simulink model "DemonstratorSimscape"  (R2020b)
settings: Solver=ode113  StartTime=0.0  StopTime=t_stop*0+20  FixedStep=1e-4
values from neighbouring files (symbols this model uses):
  brkD = 0    [main.m]
  brkI = 1e4    (= 10000)    [main.m]
  brkP = 1e5    (= 100000)    [main.m]
  d_drm = 0.5*d_drum    [main.m]
  d_shm = 0.4*d_sheave    [main.m]
  DeltaCable0 = 0    [main.m]
  Droop_scaling = 0    [main.m]
  eta_sh = 0.015    [main.m]
  filt_NUM = ones(1,200)*0.005    [main.m]
  g = 9.80665    [main.m]
  Iw = 0.5*(W.i + M.in*GB.r^2)    [main.m]
  Kp_mul = 0.3    [main.m]
  Lc0 = abs((T.ph-L.height-P.d-L.z0)*0.001)    [main.m]
  Ls1 = ((T.ph-0.5*W.pd)/1000)    [main.m]
  Ls2 = ((0.5*(T.s2+P.d)-2*P.d)/1000)    [main.m]
  M = 50e3    (= 50000)    [calcGrav.m]
  phi0_drm = -90    [main.m]
  phi0_shm = -90    [main.m]
  r_sheave = P.d*0.5    [main.m]
  s = tf('s')    [calcGrav.m]
  tau_brk = 0.001    [main.m]
  tau_em = 60e-3    (= 0.06)    [calcGrav.m]    (also in main.m)
  tau_m = tau_w/GB.r    [main.m]
  Tmax = 400e3    (= 400000)    [main.m]
  Tn_mul = 10    [main.m]
  x_drm = 0.7*r_drum    [main.m]
  x_shm = 0.7*r_sheave    [main.m]
  z0 = 0    [calcGrav.m]    (also in main.m = L.z0-P.d*0.5-P.d-P.d-L.height-T.h1-T.h2-32)
undefined symbols (not defined in the file or in its folder): C, CA, Controller_sampleTime, DiscIntNeverNeededParam, GB, L, P, Part, T, VFD_acceleration_model_factor, VFD_Adapt_factor_lower_p1458, VFD_Adapt_factor_upper_p1459, VFD_Curr_limit_var_p0641, VFD_Current_limit_p0640, VFD_Id_setp_total_r1624, VFD_Iq, VFD_Kp_n_basic_p1460, VFD_M, VFD_M_accel_T_smooth_p1517, VFD_M_lim_var_fixS_src_p1551, VFD_M_max_lower_p1521, VFD_M_max_lower_scal_p1525, VFD_M_max_up_mot_scal_p1524, VFD_M_max_upper_p1520, VFD_n_act_T_smooth_p1442, VFD_n_ctr_Kp_n_up_scal_p1461, VFD_n_ctr_Tn_n_up_sca_p1463, VFD_n_ctrl_adapt_Kp_lower_p1456, VFD_n_ctrl_adapt_Kp_upper_p1457, VFD_n_ctrl_Adpt_sig_Kp_p1455, VFD_n_ctrl_Kp_scal_p1466, VFD_n_ctrl_n_lower_p1464, VFD_n_ctrl_n_upper_p1465, VFD_n_ctrl_Tn_n_lower_p1462, VFD_n_limit_neg_p1086, VFD_n_limit_pos_p1083, VFD_n_limit_setp_p1063, VFD_n_max_p1082, VFD_n_set_filt_1_T_p1416, VFD_P_max_gen_p1531, VFD_P_max_mot_p1530, VFD_PU_I_outp_max_r0289, VFD_RFG_ramp_down_time_p1121, VFD_RFG_ramp_up_time_p1120, VFD_RFG_t_RD_scal_p1139, VFD_RFG_t_RU_scal_p1138, VSD, W, X, Y, Z
libraries: sm_lib x248, nesl_utility x128, simulink x49, pid_lib x4, cstblocks x2, simulink_extras x2
(part 1 of 10)
settings Model: Creator=pawel  LastModifiedBy=Pawel
settings SolverCC: ZeroCrossAlgorithm=Adaptive
settings DataIOCC: ReturnWorkspaceOutputs=off
settings DebuggingCC: IgnoredZcDiagnostic=none  ArithmeticOperatorsInVariantConditions=warning
settings SFSimCC: CustomCodeUndefinedFunction=UseInterfaceOnly
settings ExplorerConfigSet: InternalSimMechanicsExplorerSettings="<ExplorerConfiguration><canonicalview>planar_xy</canonicalview><AnimationSetting><BasePlaybackSpeed>1.0</BasePlaybackSpeed><PlaybackSpeedFactor>1.0</PlaybackSpeedFactor></AnimationSetting><TilePanel><TileInfo><Tiles Columns=\"1\" Count=\"1\" Rows=\"1\"><Column Weight=\"1\"/><Row Weight=\"1\"/><Tile Height=\"1\" Width=\"1\" X=\"0\" Y=\"0\"/></Tiles></TileInfo><SceneInfo><SceneViewer><BGColor><R>0.60000002384185791</R><G>0.60000002384185791</G><B>0.60000002384185791</B></BGColor><Camera><DoPerspective>off</DoPerspective><Position><X>-3.24512344704319666e-08</X><Y>5.10100123372752456</Y><Z>8.85394363287113606</Z></Position><Center><X>-3.24512344704319666e-08</X><Y>5.10100123372752456</Y><Z>2.95815624440365355e-06</Z></Center><Up><X>0</X><Y>1</Y><Z>0</Z></Up><ViewLimDist>1</ViewLimDist><YLim>5.30553002357482928</YLim><XLim>4.55308148188114892</XLim></Camera></SceneViewer></SceneInfo></TilePanel><MechEditorPanel><Cameras/><GfxPanelCameraMap/><VideoCreator><PlaybackSpeedRatio>1.0</PlaybackSpeedRatio><FrameRate>30</FrameRate><VideoFormat>Motion JPEG AVI</VideoFormat><FrameSize>auto</FrameSize></VideoCreator></MechEditorPanel></ExplorerConfiguration>"

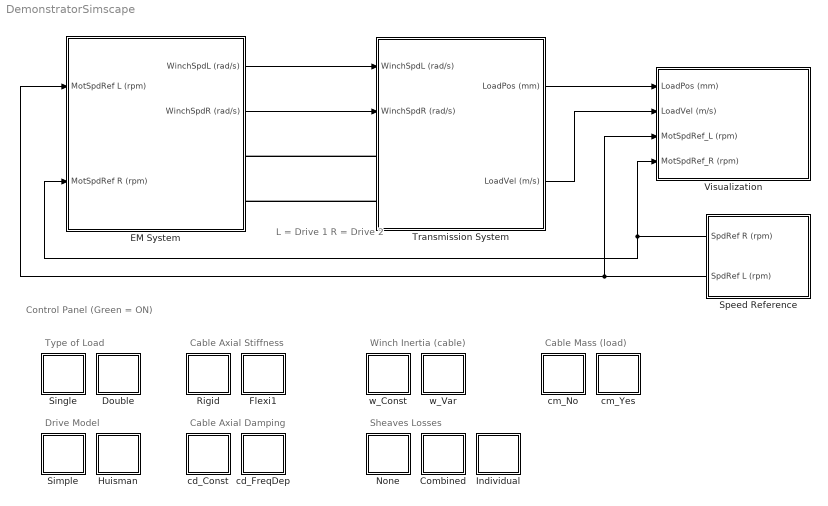
== system DemonstratorSimscape ==
  note: L = Drive 1
      | R = Drive 2
  note: Type of Load
  note: Control Panel (Green = ON)
  note: Cable Axial Stiffness
  note: Sheaves Losses
  note: Cable Mass (load)
  note: Winch Inertia (cable)
  note: Cable Axial Damping
  note: Drive Model
  Combined : Subsystem  Tag=btn_cablelosses
      settings: OpenFcn=cb_switch(gcb)
      mask Display: disp('C')
  Double : Subsystem  Tag=btn_load
      settings: OpenFcn=cb_switch(gcb)
      mask Display: disp('D')
  EM System : Subsystem
  Flexi1 : Subsystem  Tag=btn_cableflex
      settings: OpenFcn=cb_switch(gcb)
      mask Display: disp('F1')
  Huisman : Subsystem  Tag=btn_drive
      settings: OpenFcn=cb_switch(gcb)
      mask Display: disp('H')
  Individual : Subsystem  Tag=btn_cablelosses
      settings: OpenFcn=cb_switch(gcb)
      mask Display: disp('I')
  None : Subsystem  Tag=btn_cablelosses
      settings: OpenFcn=cb_switch(gcb)
      mask Display: disp('N')
  Rigid : Subsystem  Tag=btn_cableflex
      settings: OpenFcn=cb_switch(gcb)
      mask Display: disp('R')
  Simple : Subsystem  Tag=btn_drive
      settings: OpenFcn=cb_switch(gcb)
      mask Display: disp('S')
  Single : Subsystem  Tag=btn_load
      settings: OpenFcn=cb_switch(gcb)
      mask Display: disp('S')
  Speed Reference : Subsystem
  Transmission System : Subsystem
  Visualization : Subsystem
  cd_Const : Subsystem  Tag=btn_cabledamping
      settings: OpenFcn=cb_switch(gcb)
      mask Display: disp('C')
  cd_FreqDep : Subsystem  Tag=btn_cabledamping
      settings: OpenFcn=cb_switch(gcb)
      mask Display: disp('FD')
  cm_No : Subsystem  Tag=btn_cablemass
      settings: OpenFcn=cb_switch(gcb)
      mask Display: disp('NO')
  cm_Yes : Subsystem  Tag=btn_cablemass
      settings: OpenFcn=cb_switch(gcb)
      mask Display: disp('YES')
  w_Const : Subsystem  Tag=btn_winch
      settings: OpenFcn=cb_switch(gcb)
      mask Display: disp('C')
  w_Var : Subsystem  Tag=btn_winch
      settings: OpenFcn=cb_switch(gcb)
      mask Display: disp('V')
  wires:
  EM System/1(WinchSpdL (rad/s)) -> Transmission System/1(WinchSpdL (rad/s))
  EM System/2(WinchSpdR (rad/s)) -> Transmission System/2(WinchSpdR (rad/s))
  Transmission System/1(LoadPos (mm)) -> Visualization/1(LoadPos (mm))
  Transmission System/2(LoadVel (m/s)) -> Visualization/2(LoadVel (m/s))
  Speed Reference/2(SpdRef L (rpm)) -> EM System/1(MotSpdRef L (rpm)), Visualization/3(MotSpdRef_L (rpm))
  Speed Reference/1(SpdRef R (rpm)) -> EM System/2(MotSpdRef R (rpm)), Visualization/4(MotSpdRef_R (rpm))
  connections:
  Transmission System/LConn1 -- EM System/RConn1
  Transmission System/LConn2 -- EM System/RConn2

== system DemonstratorSimscape/Combined ==

== system DemonstratorSimscape/Double ==

== system DemonstratorSimscape/EM System ==
  MotSpdRef L (rpm) : Inport  SampleTime=C.ts
  MotSpdRef R (rpm) : Inport  Port=2  SampleTime=C.ts
  Belt-Cable Spool1 : sm_lib/Belts and Cables/Belt-Cable Spool  PitchRadius=W.d*0.5  PitchRadiusUnits=mm  SenseSpoolAngleA=off  SenseFleetAngleA=off
      settings: SourceProductBaseCode=MS
  Belt-Cable Spool2 : sm_lib/Belts and Cables/Belt-Cable Spool  PitchRadius=W.d*0.5  PitchRadiusUnits=mm  SenseSpoolAngleA=off  SenseFleetAngleA=off
      settings: SourceProductBaseCode=MS
  BrakeL_OFF : FromWorkspace  VariableName=BrakeOffL_inp  Interpolate=off  OutputAfterFinalValue=Holding final value
  BrakeR_OFF : FromWorkspace  VariableName=BrakeOffR_inp  Interpolate=off  OutputAfterFinalValue=Holding final value
  Constant : Constant
  Drives : Subsystem
  Motor Winch Left : Subsystem
  Motor Winch Right : Subsystem
  Product : Product
  Product1 : Product
  Winch Left (yellow) : Subsystem
      mask Display: image('sm_cable_drive_right_angle_winch_IMAGE.png');
  Winch Right (blue) : Subsystem
      mask Display: image('sm_cable_drive_right_angle_winch_IMAGE.png');
  swBrake : ManualSwitch  CurrentSetting=0
  swBrake1 : ManualSwitch
  RWinch : PMIOPort  Side=Right
  LWinch : PMIOPort  Port=2  Side=Right
  WinchSpdL (rad/s) : Outport  VectorParamsAs1DForOutWhenUnconnected=off
  WinchSpdR (rad/s) : Outport  Port=2  VectorParamsAs1DForOutWhenUnconnected=off
  tag scope: BrakeL_OFF=global, BrakeR_OFF=global, MotSpd_L_rpm=global, MotSpd_R_rpm=global, MotTrqRef_L_Nm=global, MotTrqRef_R_Nm=global, MotTrq_L_Nm=global, MotTrq_R_Nm=global
  wires:
  Motor Winch Left/2(theta [deg]) -> Winch Left (yellow)/1(theta winch (deg))
  Winch Right (blue)/1(r_winch (mm)) -> Motor Winch Right/2(winch radius)
  Motor Winch Right/2(theta [deg]) -> Winch Right (blue)/1(theta winch (deg))
  Motor Winch Left/3(WinchSpd (rad/s)) -> WinchSpdL (rad/s)/1
  Motor Winch Right/3(WinchSpd (rad/s)) -> WinchSpdR (rad/s)/1
  Drives/1(TrqRefL (Nm)) -> Motor Winch Left/1(MotTrqRef (Nm)), Product/2
  Motor Winch Right/1(MotSpd (rpm)) -> Drives/4(SpdR (rpm)), [MotSpd_R_rpm]
  Motor Winch Left/1(MotSpd (rpm)) -> Drives/1(SpdL (rpm)), [MotSpd_L_rpm]
  Drives/2(TrqRefR (Nm)) -> Product1/2, Motor Winch Right/1(MotTrqRef (Nm))
  Motor Winch Left/4(MotTrq (Nm)) -> [MotTrq_L_Nm]
  Motor Winch Right/4(MotTrq) -> [MotTrq_R_Nm]
  Winch Left (yellow)/1(r_winch (mm)) -> Motor Winch Left/2(winch radius)
  MotSpdRef L (rpm)/1 -> Drives/2(SpdRefL (rpm))
  MotSpdRef R (rpm)/1 -> Drives/3(SpdRefR (rpm))
  Product/1 -> [MotTrqRef_L_Nm]
  Product1/1 -> [MotTrqRef_R_Nm]
  swBrake/1 -> Motor Winch Left/3(Brake), Product/1, [BrakeL_OFF]
  BrakeL_OFF/1 -> swBrake/1
  Constant/1 -> swBrake1/1, swBrake/2
  BrakeR_OFF/1 -> swBrake1/2
  swBrake1/1 -> [BrakeR_OFF], Motor Winch Right/3(Brake), Product1/1
  connections:
  Belt-Cable Spool1/LConn1 -- Winch Right (blue)/LConn1
  RWinch/RConn1 -- Belt-Cable Spool1/RConn1
  Winch Right (blue)/RConn1 -- Motor Winch Right/RConn1
  Belt-Cable Spool2/LConn1 -- Winch Left (yellow)/LConn1
  Winch Left (yellow)/RConn1 -- Motor Winch Left/RConn1
  LWinch/RConn1 -- Belt-Cable Spool2/RConn1

== system DemonstratorSimscape/Flexi1 ==

== system DemonstratorSimscape/Huisman ==

== system DemonstratorSimscape/Individual ==

== system DemonstratorSimscape/None ==

== system DemonstratorSimscape/Rigid ==

== system DemonstratorSimscape/Simple ==

== system DemonstratorSimscape/Single ==

== system DemonstratorSimscape/Speed Reference ==
  Add : Sum
  Gain : Gain
  Gain1 : Gain
  Manual Switch : ManualSwitch
  Manual Switch1 : ManualSwitch
  SpdRef_L_rpm : FromWorkspace  VariableName=SpdRefL_inp  OutputAfterFinalValue=Holding final value
  SpdRef_R_rpm : FromWorkspace  VariableName=SpdRefR_inp  OutputAfterFinalValue=Holding final value
  Step : Step  After=1000  SampleTime=0
  Step1 : Step  Time=10  After=-1000  SampleTime=0
  SpdRef R (rpm) : Outport  VectorParamsAs1DForOutWhenUnconnected=off
  SpdRef L (rpm) : Outport  Port=2  VectorParamsAs1DForOutWhenUnconnected=off
  wires:
  SpdRef_L_rpm/1 -> Gain/1
  SpdRef_R_rpm/1 -> Gain1/1
  Step1/1 -> Add/2
  Step/1 -> Add/1
  Add/1 -> Manual Switch1/1, Manual Switch/1
  Gain/1 -> Manual Switch/2
  Gain1/1 -> Manual Switch1/2
  Manual Switch1/1 -> SpdRef R (rpm)/1
  Manual Switch/1 -> SpdRef L (rpm)/1

== system DemonstratorSimscape/Transmission System ==
  WinchSpdL (rad/s) : Inport
  WinchSpdR (rad/s) : Inport  Port=2
  Anchor and Load : Subsystem
  Mechanism Configuration1 : sm_lib/Utilities/Mechanism Configuration  UniformGravity=Constant  GravityVector=[0 -g 0]  GravityVectorUnits=m/s^2  GravityUnits=m/s^2  LinearizationDelta=0.001  JointModeTransitionNonlinearIterations=2
  Roof Pulley Set : Subsystem
  Solver Configuration : nesl_utility/Solver Configuration  PhysicalDomain=network_engine_domain  SubClassName=solver  LeftPortType=input  RightPortType=generic  Tones=[]  Harmonics=[]  SimulateNoise=off  Profile=off  UseLocalSampling=off  EnableSwitchedLinearOptims=on  FrequencyDomain=off  UseCCode=off  RelTol=0.001  AbsTol=1e-06  MinStep=1e-09  ToWorkspace=off  RevertToSquareIcSolve=off  NumHomotopyIterations=100  PhasorMode=off  PhasorModeNumHarmonics=1  DoDC=off  ResidualTolerance=1e-09  UseLocalSolver=off  LocalSolverChoice=NE_PARTITIONING_ADVANCER  LocalSolverSampleTime=0.001  DoFixedCost=off  MaxNonlinIter=30  MaxModeIter=2  ComputeImpulses=off  ImpulseIterations=2  LinearAlgebra=auto  EquationFormulation=NE_TIME_EF  DelaysMemoryBudget=10240  AutomaticFiltering=on  FilteringTimeConstant=0.001  PartitionStorageMethod=AS_NEEDED  PartitionMemoryBudget=1024  PartitionMethod=FAST
  Tower structure : Subsystem
  World Frame : sm_lib/Frames and Transforms/World Frame
  RWinch : PMIOPort  Side=Left
  LWinch : PMIOPort  Port=2  Side=Left
  LoadPos (mm) : Outport
  LoadVel (m/s) : Outport  Port=2
  wires:
  Roof Pulley Set/1(w7) -> Anchor and Load/1(w7)
  Roof Pulley Set/2(w6) -> Anchor and Load/2(w6)
  Roof Pulley Set/3(w4) -> Anchor and Load/3(w4)
  Roof Pulley Set/5(w1) -> Anchor and Load/5(w1)
  Anchor and Load/1(LoadPos (mm)) -> LoadPos (mm)/1
  Roof Pulley Set/4(w2) -> Anchor and Load/4(w2)
  Anchor and Load/2(LoadVel (m/s)) -> LoadVel (m/s)/1
  WinchSpdL (rad/s)/1 -> Anchor and Load/6(wL)
  WinchSpdR (rad/s)/1 -> Anchor and Load/7(wR)
  connections:
  Solver Configuration/RConn1 -- Tower structure/LConn1 -- Mechanism Configuration1/RConn1 -- Roof Pulley Set/LConn1 -- World Frame/RConn1
  Roof Pulley Set/RConn2 -- Anchor and Load/LConn3
  Anchor and Load/LConn1 -- Roof Pulley Set/RConn1
  Roof Pulley Set/RConn3 -- Anchor and Load/LConn4
  Roof Pulley Set/RConn5 -- Anchor and Load/LConn5
  Anchor and Load/LConn2 -- Roof Pulley Set/RConn4
  Roof Pulley Set/LConn2 -- RWinch/RConn1
  Roof Pulley Set/LConn3 -- LWinch/RConn1

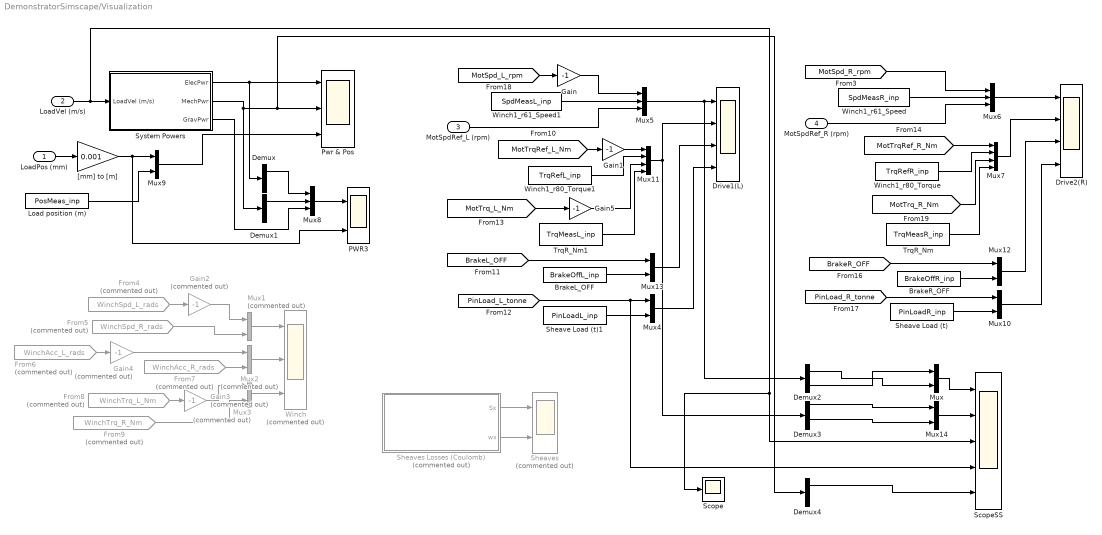
== system DemonstratorSimscape/Visualization ==
  LoadPos (mm) : Inport
  LoadVel (m/s) : Inport  Port=2
  MotSpdRef_L (rpm) : Inport  Port=3
  MotSpdRef_R (rpm) : Inport  Port=4
  BrakeL_OFF : FromWorkspace  VariableName=BrakeOffL_inp  Interpolate=off  OutputAfterFinalValue=Holding final value
  BrakeR_OFF : FromWorkspace  VariableName=BrakeOffR_inp  Interpolate=off  OutputAfterFinalValue=Holding final value
  Demux : Demux  Outputs=2
  Demux1 : Demux  Outputs=2
  Demux2 : Demux  Outputs=3
  Demux3 : Demux
  Demux4 : Demux  Outputs=2
  Drive1(L) : Scope  NumInputPorts=4
  Drive2(R) : Scope  NumInputPorts=4
  From4 : From  Commented=on  GotoTag=WinchSpd_L_rads  TagVisibility=global
  From5 : From  Commented=on  GotoTag=WinchSpd_R_rads  TagVisibility=global
  From6 : From  Commented=on  GotoTag=WinchAcc_L_rads  TagVisibility=global
  From7 : From  Commented=on  GotoTag=WinchAcc_R_rads  TagVisibility=global
  From8 : From  Commented=on  GotoTag=WinchTrq_L_Nm  TagVisibility=global
  From9 : From  Commented=on  GotoTag=WinchTrq_R_Nm  TagVisibility=global
  Gain : Gain  Gain=-1
  Gain1 : Gain  Gain=-1
  Gain2 : Gain  Commented=on  Gain=-1
  Gain3 : Gain  Commented=on  Gain=-1
  Gain4 : Gain  Commented=on  Gain=-1
  Gain5 : Gain  Gain=-1
  Load position (m) : FromWorkspace  VariableName=PosMeas_inp  Interpolate=off  OutputAfterFinalValue=Holding final value
  Mux{,4,9..10,12..14} (7 alike) : Mux  Inputs=2
  Mux1 : Mux  Commented=on  Inputs=2
  Mux11 : Mux
  Mux2 : Mux  Commented=on  Inputs=2
  Mux3 : Mux  Commented=on  Inputs=2
  Mux5 : Mux  Inputs=3
  Mux6 : Mux  Inputs=3
  Mux7 : Mux
  Mux8 : Mux  Inputs=3
  PWR3 : Scope  NumInputPorts=2
  Pwr & Pos : Scope  NumInputPorts=3
  Scope : Scope
  ScopeSS : Scope  NumInputPorts=5
  Sheave Load (t) : FromWorkspace  VariableName=PinLoadR_inp  Interpolate=off  OutputAfterFinalValue=Holding final value
  Sheave Load (t)1 : FromWorkspace  VariableName=PinLoadL_inp  Interpolate=off  OutputAfterFinalValue=Holding final value
  Sheaves : Scope  Commented=on  NumInputPorts=2
  Sheaves Losses (Coulomb) : Subsystem  Commented=on
  System Powers : Subsystem
  TrqR_Nm : FromWorkspace  VariableName=TrqMeasR_inp  OutputAfterFinalValue=Holding final value
  TrqR_Nm1 : FromWorkspace  VariableName=TrqMeasL_inp  OutputAfterFinalValue=Holding final value
  Winch : Scope  Commented=on  NumInputPorts=3
  Winch1_r61_Speed : FromWorkspace  VariableName=SpdMeasR_inp  Interpolate=off  OutputAfterFinalValue=Holding final value
  Winch1_r61_Speed1 : FromWorkspace  VariableName=SpdMeasL_inp  Interpolate=off  OutputAfterFinalValue=Holding final value
  Winch1_r80_Torque : FromWorkspace  VariableName=TrqRefR_inp  Interpolate=off  OutputAfterFinalValue=Holding final value
  Winch1_r80_Torque1 : FromWorkspace  VariableName=TrqRefL_inp  Interpolate=off  OutputAfterFinalValue=Holding final value
  "[mm] to [m]" : Gain  Gain=0.001
  wires:
  Mux1/1 -> Winch/1
  Mux2/1 -> Winch/2
  Mux3/1 -> Winch/3
  From4/1 -> Gain2/1
  From5/1 -> Mux1/2
  From6/1 -> Gain4/1
  From7/1 -> Mux2/2
  From8/1 -> Gain3/1
  From9/1 -> Mux3/2
  Gain2/1 -> Mux1/1
  Gain3/1 -> Mux3/1
  Gain4/1 -> Mux2/1
  "[mm] to [m]"/1 -> PWR3/2, Mux9/1
  MotSpdRef_R (rpm)/1 -> Mux6/3
  [MotTrqRef_R_Nm] -> Mux7/1
  Winch1_r61_Speed/1 -> Mux6/2
  Winch1_r80_Torque/1 -> Mux7/2
  [MotSpd_R_rpm] -> Mux6/1
  Load position (m)/1 -> Mux9/2
  Sheave Load (t)/1 -> Mux10/2
  [PinLoad_R_tonne] -> Mux10/1
  [MotTrq_R_Nm] -> Mux7/3
  TrqR_Nm/1 -> Mux7/4
  Mux6/1 -> Drive2(R)/1
  Mux7/1 -> Drive2(R)/2
  Mux10/1 -> Drive2(R)/4
  Mux4/1 -> Drive1(L)/4
  Mux11/1 -> Demux3/1, Drive1(L)/2
  Mux5/1 -> Demux2/1, Drive1(L)/1
  TrqR_Nm1/1 -> Mux11/4
  [MotTrq_L_Nm] -> Gain5/1
  [PinLoad_L_tonne] -> ScopeSS/4, Mux4/1
  Sheave Load (t)1/1 -> Mux4/2
  [MotSpd_L_rpm] -> Gain/1
  Winch1_r80_Torque1/1 -> Mux11/2
  Winch1_r61_Speed1/1 -> Mux5/2
  [MotTrqRef_L_Nm] -> Gain1/1
  MotSpdRef_L (rpm)/1 -> Mux5/3
  Mux12/1 -> Drive2(R)/3
  Mux13/1 -> Drive1(L)/3
  [BrakeL_OFF] -> Mux13/1
  BrakeL_OFF/1 -> Mux13/2
  [BrakeR_OFF] -> Mux12/1
  BrakeR_OFF/1 -> Mux12/2
  Gain/1 -> Mux5/1
  Gain1/1 -> Mux11/1
  Gain5/1 -> Mux11/3
  LoadPos (mm)/1 -> "[mm] to [m]"/1
  Mux9/1 -> Pwr & Pos/3
  System Powers/1(ElecPwr) -> Demux/1, Pwr & Pos/1
  System Powers/2(MechPwr) -> Demux1/1, Demux4/1, Pwr & Pos/2
  LoadVel (m/s)/1 -> Scope/1, ScopeSS/3, System Powers/1(LoadVel (m/s))
  Mux8/1 -> PWR3/1
  Demux/1 -> Mux8/1
  Demux1/1 -> Mux8/2
  System Powers/3(GravPwr) -> Mux8/3
  Sheaves Losses (Coulomb)/1(Sx) -> Sheaves/1
  Sheaves Losses (Coulomb)/2(wx) -> Sheaves/2
  Mux/1 -> ScopeSS/1
  Mux14/1 -> ScopeSS/2
  Demux4/1 -> ScopeSS/5
  Demux2/3 -> Mux/1
  Demux2/1 -> Mux/2
  Demux3/1 -> Mux14/1
  Demux3/3 -> Mux14/2

== system DemonstratorSimscape/cd_Const ==

== system DemonstratorSimscape/cd_FreqDep ==

== system DemonstratorSimscape/cm_No ==

== system DemonstratorSimscape/cm_Yes ==

== system DemonstratorSimscape/w_Const ==

== system DemonstratorSimscape/w_Var ==

== system DemonstratorSimscape/EM System/Drives ==
  SpdL (rpm) : Inport
  SpdRefL (rpm) : Inport  Port=2
  SpdRefR (rpm) : Inport  Port=3
  SpdR (rpm) : Inport  Port=4
  Add : Sum
  Bus Selector : BusSelector  Commented=on  OutputSignals=signal1.[r1468] Speed Controller P-gain effective,signal1.[r1469] Speed Controller integral time effective,signal1.[r1480] Speed Controller PI torque Output,signal1.[r1481] Speed Controller P torque Output,signal1.[r1482] Speed Controller I torque Output,signal1.[r1508] Torque setpoint before supplementary torque,signal1.[r1516] Supplementary torque and acceleration torque
  Bus Selector1 : BusSelector  Commented=on  OutputSignals=signal1.[r1468] Speed Controller P-gain effective,signal1.[r1469] Speed Controller integral time effective,signal1.[r1480] Speed Controller PI torque Output,signal1.[r1481] Speed Controller P torque Output,signal1.[r1482] Speed Controller I torque Output,signal1.[r1508] Torque setpoint before supplementary torque,signal1.[r1516] Supplementary torque and acceleration torque
  Constant : Constant
  Constant1 : Constant
  DIAG1 : Scope  Commented=on  NumInputPorts=7
  DIAG2 : Scope  Commented=on  NumInputPorts=7
  Gain1 : Gain  Gain=-1
  Gain2 : Gain  Gain=-1
  Gain5 : Gain  Gain=-1
  PLC and Drive Logic Rev3 : Subsystem  AncestorBlock=Control_Library_Rev3/PLC and Drive Logic
  SWTL : ManualSwitch  CurrentSetting=0
  SWTR : ManualSwitch  CurrentSetting=0
  Simple Drive Model : Subsystem  Commented=on
  Simple Drive Model1 : Subsystem  Commented=on
  Step : Step  Time=5  Before=tau_m  After=1.5*tau_m  SampleTime=0
  Step2 : Step  Time=5.2  After=-0.5*tau_m  SampleTime=0
  Winch1_r80_Torque : FromWorkspace  VariableName=TrqRefR_inp  OutputAfterFinalValue=Holding final value
  Winch1_r80_Torque1 : FromWorkspace  VariableName=TrqRefL_inp  OutputAfterFinalValue=Holding final value
  swTrqRefL : ManualSwitch
  swTrqRefR : ManualSwitch
  TrqRefL (Nm) : Outport
  TrqRefR (Nm) : Outport  Port=2
  wires:
  Constant/1 -> PLC and Drive Logic Rev3/3(HMI Motor 1 Start Test [0...1]), PLC and Drive Logic Rev3/5(HMI Motor 2 Start Test [0...1])
  Constant1/1 -> PLC and Drive Logic Rev3/7(WAB Mode)
  SWTL/1 -> swTrqRefL/1
  swTrqRefL/1 -> TrqRefL (Nm)/1
  SWTR/1 -> swTrqRefR/1
  swTrqRefR/1 -> TrqRefR (Nm)/1
  PLC and Drive Logic Rev3/4(M2 [r0079] M_set total (Torque setpoint [Nm])) -> SWTR/2
  Winch1_r80_Torque1/1 -> Gain2/1
  PLC and Drive Logic Rev3/1(M1 [r0079] M_set total (Torque setpoint [Nm])) -> SWTL/2
  Gain5/1 -> PLC and Drive Logic Rev3/8(WAB Motor 1 Speed_Controller Setpoint (r1438))
  SpdL (rpm)/1 -> PLC and Drive Logic Rev3/2(Motor 1 Actual Speed (rpm)), Simple Drive Model/1(Spd_L)
  SpdRefL (rpm)/1 -> Gain5/1, Simple Drive Model/2(SpdRef_L)
  SpdR (rpm)/1 -> PLC and Drive Logic Rev3/6(Motor 2 Actual Speed (rpm)), Simple Drive Model/3(Spd_R)
  SpdRefR (rpm)/1 -> PLC and Drive Logic Rev3/9(WAB Motor 2 Speed_Controller Setpoint (r1438)), Simple Drive Model/4(SpdRef_R)
  Bus Selector/1 -> DIAG1/1  "<[r1468] Speed Controller P-gain effective>"
  Bus Selector/2 -> DIAG1/2  "<[r1469] Speed Controller integral time effective>"
  Bus Selector/3 -> DIAG1/3  "<[r1480] Speed Controller PI torque Output>"
  Bus Selector/4 -> DIAG1/4  "<[r1481] Speed Controller P torque Output>"
  Bus Selector/5 -> DIAG1/5  "<[r1482] Speed Controller I torque Output>"
  Bus Selector/6 -> DIAG1/6  "<[r1508] Torque setpoint before supplementary torque>"
  Bus Selector/7 -> DIAG1/7  "<[r1516] Supplementary torque and acceleration torque>"
  Bus Selector1/1 -> DIAG2/1  "<[r1468] Speed Controller P-gain effective>"
  Bus Selector1/2 -> DIAG2/2  "<[r1469] Speed Controller integral time effective>"
  Bus Selector1/3 -> DIAG2/3  "<[r1480] Speed Controller PI torque Output>"
  Bus Selector1/4 -> DIAG2/4  "<[r1481] Speed Controller P torque Output>"
  Bus Selector1/5 -> DIAG2/5  "<[r1482] Speed Controller I torque Output>"
  Bus Selector1/6 -> DIAG2/6  "<[r1508] Torque setpoint before supplementary torque>"
  Bus Selector1/7 -> DIAG2/7  "<[r1516] Supplementary torque and acceleration torque>"
  PLC and Drive Logic Rev3/3(Motor 1 Diagnostics Bus) -> Bus Selector/1
  PLC and Drive Logic Rev3/5(Motor 2 Diagnostics Bus) -> Bus Selector1/1
  Simple Drive Model/2(TrqSat_R) -> SWTR/1
  Step/1 -> Add/1
  Step2/1 -> Add/2
  Add/1 -> swTrqRefR/2, Gain1/1
  Gain1/1 -> swTrqRefL/2
  Simple Drive Model/1(TrqSat_L) -> SWTL/1

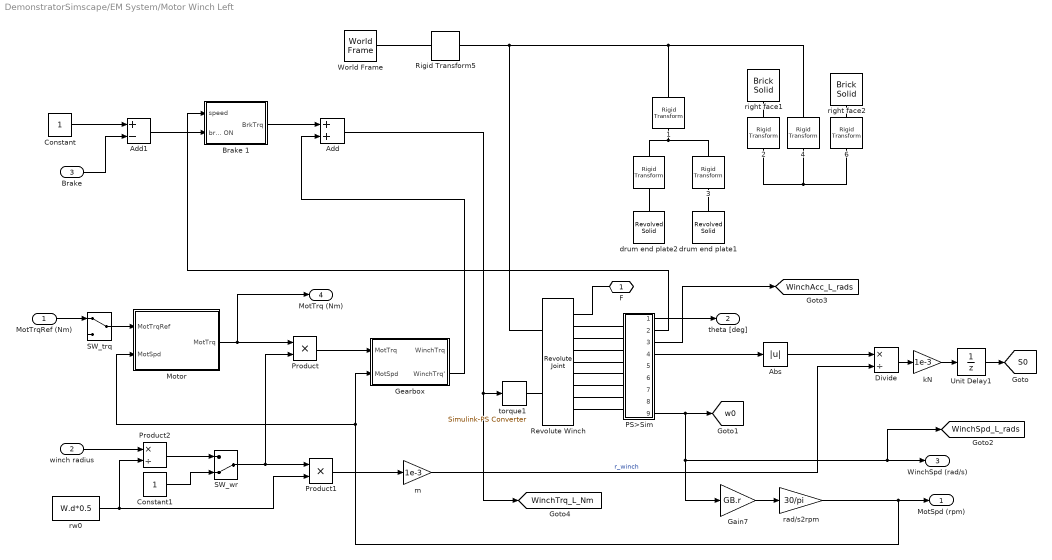
== system DemonstratorSimscape/EM System/Motor Winch Left ==
  MotTrqRef (Nm) : Inport
  winch radius : Inport  Port=2
  Brake : Inport  Port=3
  " " : sm_lib/Frames and Transforms/Rigid Transform  TranslationMethod=Cartesian  TranslationStandardOffset=0  TranslationLengthUnit=mm  TranslationStandardAxis=+Z  TranslationCartesianOffset=[0 0 -W.pds*.5]  TranslationROffset=0  TranslationROffsetUnits=m  TranslationZOffset=0  TranslationZOffsetUnits=m  TranslationThetaOffset=0  TranslationThetaOffsetUnits=deg  RotationMethod=StandardAxis  RotationAngleUnits=deg  RotationStandardAxis=-X  RotationAngle=90  RotationArbitraryAxis=[1 0 0]  FollAlignAxisA=+X  BaseAlignAxisA=+Y  FollAlignAxisB=+Y  BaseAlignAxisB=+Z  RotationSequenceAxes=FollowerAxes  RotationSequence=XYX  RotationSequenceAngles=[0 0 0]  RotationSequenceAnglesUnits=deg  RotationMatrix=[1 0 0; 0 1 0; 0 0 1]
  " 1" : sm_lib/Frames and Transforms/Rigid Transform  TranslationMethod=Cartesian  TranslationStandardOffset=0  TranslationLengthUnit=mm  TranslationStandardAxis=+Z  TranslationCartesianOffset=[0 0 W.w*0.5+W.pds*0.5]  TranslationROffset=0  TranslationROffsetUnits=m  TranslationZOffset=0  TranslationZOffsetUnits=m  TranslationThetaOffset=0  TranslationThetaOffsetUnits=deg  RotationMethod=StandardAxis  RotationAngleUnits=deg  RotationStandardAxis=+X  RotationAngle=90  RotationArbitraryAxis=[1 0 0]  FollAlignAxisA=+X  BaseAlignAxisA=+Y  FollAlignAxisB=+Y  BaseAlignAxisB=+Z  RotationSequenceAxes=FollowerAxes  RotationSequence=XYX  RotationSequenceAngles=[0 0 0]  RotationSequenceAnglesUnits=deg  RotationMatrix=[1 0 0; 0 1 0; 0 0 1]
  " 2" : sm_lib/Frames and Transforms/Rigid Transform  TranslationMethod=Cartesian  TranslationStandardOffset=0  TranslationLengthUnit=mm  TranslationStandardAxis=+Z  TranslationCartesianOffset=[0 -W.pd*.25 -W.pds]  TranslationROffset=0  TranslationROffsetUnits=m  TranslationZOffset=0  TranslationZOffsetUnits=m  TranslationThetaOffset=0  TranslationThetaOffsetUnits=deg  RotationMethod=ArbitraryAxis  RotationAngleUnits=deg  RotationStandardAxis=+X  RotationAngle=90  RotationArbitraryAxis=[1 0 0]  FollAlignAxisA=+X  BaseAlignAxisA=+Y  FollAlignAxisB=+Y  BaseAlignAxisB=+Z  RotationSequenceAxes=FollowerAxes  RotationSequence=XYX  RotationSequenceAngles=[0 0 0]  RotationSequenceAnglesUnits=deg  RotationMatrix=[1 0 0; 0 1 0; 0 0 1]
  " 3" : sm_lib/Frames and Transforms/Rigid Transform  TranslationMethod=Cartesian  TranslationStandardOffset=0  TranslationLengthUnit=mm  TranslationStandardAxis=+Z  TranslationCartesianOffset=[0 -W.w -W.pds*.5]  TranslationROffset=0  TranslationROffsetUnits=m  TranslationZOffset=0  TranslationZOffsetUnits=m  TranslationThetaOffset=0  TranslationThetaOffsetUnits=deg  RotationMethod=StandardAxis  RotationAngleUnits=deg  RotationStandardAxis=+X  RotationAngle=90  RotationArbitraryAxis=[1 0 0]  FollAlignAxisA=+X  BaseAlignAxisA=+Y  FollAlignAxisB=+Y  BaseAlignAxisB=+Z  RotationSequenceAxes=FollowerAxes  RotationSequence=XYX  RotationSequenceAngles=[0 0 0]  RotationSequenceAnglesUnits=deg  RotationMatrix=[1 0 0; 0 1 0; 0 0 1]
  " 4" : sm_lib/Frames and Transforms/Rigid Transform  TranslationMethod=Cartesian  TranslationStandardOffset=0  TranslationLengthUnit=mm  TranslationStandardAxis=+Z  TranslationCartesianOffset=[0 0 -W.w*.5]  TranslationROffset=0  TranslationROffsetUnits=m  TranslationZOffset=0  TranslationZOffsetUnits=m  TranslationThetaOffset=0  TranslationThetaOffsetUnits=deg  RotationMethod=None  RotationAngleUnits=deg  RotationStandardAxis=+Z  RotationAngle=90  RotationArbitraryAxis=[1 0 0]  FollAlignAxisA=+X  BaseAlignAxisA=+Y  FollAlignAxisB=+Y  BaseAlignAxisB=+Z  RotationSequenceAxes=FollowerAxes  RotationSequence=XYX  RotationSequenceAngles=[0 0 0]  RotationSequenceAnglesUnits=deg  RotationMatrix=[1 0 0; 0 1 0; 0 0 1]
  " 6" : sm_lib/Frames and Transforms/Rigid Transform  TranslationMethod=Cartesian  TranslationStandardOffset=0  TranslationLengthUnit=mm  TranslationStandardAxis=+Z  TranslationCartesianOffset=[0 -W.pd*.25 W.w+W.pds*2]  TranslationROffset=0  TranslationROffsetUnits=m  TranslationZOffset=0  TranslationZOffsetUnits=m  TranslationThetaOffset=0  TranslationThetaOffsetUnits=deg  RotationMethod=ArbitraryAxis  RotationAngleUnits=deg  RotationStandardAxis=+X  RotationAngle=90  RotationArbitraryAxis=[1 0 0]  FollAlignAxisA=+X  BaseAlignAxisA=+Y  FollAlignAxisB=+Y  BaseAlignAxisB=+Z  RotationSequenceAxes=FollowerAxes  RotationSequence=XYX  RotationSequenceAngles=[0 0 0]  RotationSequenceAnglesUnits=deg  RotationMatrix=[1 0 0; 0 1 0; 0 0 1]
  Abs : Abs
  Add : Sum
  Add1 : Sum  Inputs=+-
  Brake 1 : Subsystem
  Constant : Constant
  Constant1 : Constant
  Divide : Product  Inputs=*/
  Gain7 : Gain  Gain=GB.r
  Gearbox : Subsystem
  Motor : Subsystem
  PS>Sim : Subsystem
  Product : Product
  Product1 : Product
  Product2 : Product  Inputs=*/
  Revolute Winch : sm_lib/Joints/Revolute Joint  JointMode=Normal  SenseConstraintForce=on  SenseConstraintForceX=off  SenseConstraintForceY=off  SenseConstraintForceZ=off  SenseConstraintTorque=on  SenseConstraintTorqueX=off  SenseConstraintTorqueY=off  SenseConstraintTorqueZ=off  SenseTotalForce=on  SenseTotalForceX=off  SenseTotalForceY=off  SenseTotalForceZ=off  SenseTotalTorque=on  SenseTotalTorqueX=off  SenseTotalTorqueY=off  SenseTotalTorqueZ=off  CompositeWrenchDir=FollowerOnBase  CompositeWrenchFrame=BaseFrame  EquilibriumPosition=0  EquilibriumPositionUnits=deg  SpringStiffness=0  SpringStiffnessUnits=N*m/deg  DampingCoefficient=b_winch  DampingCoefficientUnits=N*m/(deg/s)  TorqueActuationMode=InputTorque  MotionActuationMode=ComputedMotion  SensePosition=on  SenseVelocity=on  SenseAcceleration=on  SenseTorqueForce=on  SenseLowerLimitTorqueForce=off  SenseUpperLimitTorqueForce=off  LowerLimitSpecify=off  LowerLimitBound=-90  LowerLimitBoundUnits=deg  LowerLimitStiffness=1e4  LowerLimitStiffnessUnits=N*m/deg  LowerLimitDamping=10  LowerLimitDampingUnits=N*m/(deg/s)  LowerLimitTransitionRegionWidth=0.1  LowerLimitTransitionRegionWidthUnits=deg  UpperLimitSpecify=off  UpperLimitBound=90  UpperLimitBoundUnits=deg  UpperLimitStiffness=1e4  UpperLimitStiffnessUnits=N*m/deg  UpperLimitDamping=10  UpperLimitDampingUnits=N*m/(deg/s)  UpperLimitTransitionRegionWidth=0.1  UpperLimitTransitionRegionWidthUnits=deg  PositionTargetSpecify=off  PositionTargetPriority=High  PositionTargetValue=0  PositionTargetValueUnits=deg  VelocityTargetSpecify=on  VelocityTargetPriority=High  VelocityTargetValue=w0_winch  VelocityTargetValueUnits=deg/s
  Rigid Transform5 : sm_lib/Frames and Transforms/Rigid Transform  TranslationMethod=Cartesian  TranslationStandardOffset=0  TranslationLengthUnit=mm  TranslationStandardAxis=+Z  TranslationCartesianOffset="[-(0.5*T.s2+0.5*W.d)  W.pd*.5  0]"  TranslationROffset=0  TranslationROffsetUnits=m  TranslationZOffset=0  TranslationZOffsetUnits=m  TranslationThetaOffset=0  TranslationThetaOffsetUnits=deg  RotationMethod=StandardAxis  RotationAngleUnits=deg  RotationStandardAxis=+Y  RotationAngle=0  RotationArbitraryAxis=[0 0 1]  FollAlignAxisA=+X  BaseAlignAxisA=+Y  FollAlignAxisB=+Y  BaseAlignAxisB=+Z  RotationSequenceAxes=FollowerAxes  RotationSequence=XYX  RotationSequenceAngles=[0 0 0]  RotationSequenceAnglesUnits=deg  RotationMatrix=[1 0 0; 0 1 0; 0 0 1]
  SW_trq : ManualSwitch
  SW_wr : ManualSwitch  CurrentSetting=0
  Unit Delay1 : UnitDelay  InitialCondition=130.83  SampleTime=-1  HasFrameUpgradeWarning=on
  World Frame : sm_lib/Frames and Transforms/World Frame
  drum end plate1 : sm_lib/Body Elements/Revolved Solid  GraphicAmbientColor=[0.15 0.15 0.15 1.0]  BasedOnType=Density  CenterOfMass=[0 0 0]  CenterOfMassUnits=m  GraphicDiffuseColor=[1.0 0.2 0.2]  ExportConvexHullGeometry=off  Density=0  DensityUnits=g/cm^3  DoExposeReferenceFrame=on  GraphicEmissiveColor=[0.0 0.0 0.0 1.0]  ExportEntireGeometry=off  SerializedFrames=<Frames/>  MarkerShape=Sphere  MarkerSize=10  GraphicType=FromGeometry  InertiaType=CalculateFromGeometry  Mass=1  MassUnits=kg  MomentsOfInertia=[1 1 1]  MomentsOfInertiaUnits=kg*m^2  GraphicOpacity=1.0  ProductsOfInertia=[0 0 0]  ProductsOfInertiaUnits=kg*m^2  RevolutionCrossSection=[W.pd*.5 0; W.pd*.5 W.pds; W.pd*0.05 W.pds; W.pd*.05 0]  RevolutionCrossSectionUnits=mm  RevolutionAngle=180  RevolutionAngleUnits=deg  RevolutionExtent=Full  GraphicShininess=75  GraphicSpecularColor=[0.5 0.5 0.5 1.0]  GraphicVisPropType=SimpleVisualProperties
  drum end plate2 : sm_lib/Body Elements/Revolved Solid  GraphicAmbientColor=[0.15 0.15 0.15 1.0]  BasedOnType=Density  CenterOfMass=[0 0 0]  CenterOfMassUnits=m  GraphicDiffuseColor=[0.0 0.8 0.0]  ExportConvexHullGeometry=off  Density=0  DensityUnits=g/cm^3  DoExposeReferenceFrame=on  GraphicEmissiveColor=[0.0 0.0 0.0 1.0]  ExportEntireGeometry=off  SerializedFrames=<Frames/>  MarkerShape=Sphere  MarkerSize=10  GraphicType=FromGeometry  InertiaType=CalculateFromGeometry  Mass=1  MassUnits=kg  MomentsOfInertia=[1 1 1]  MomentsOfInertiaUnits=kg*m^2  GraphicOpacity=1.0  ProductsOfInertia=[0 0 0]  ProductsOfInertiaUnits=kg*m^2  RevolutionCrossSection=[W.pd*.5 0; W.pd*.5 W.pds; W.pd*0.05 W.pds; W.pd*.05 0]  RevolutionCrossSectionUnits=mm  RevolutionAngle=180  RevolutionAngleUnits=deg  RevolutionExtent=Full  GraphicShininess=75  GraphicSpecularColor=[0.5 0.5 0.5 1.0]  GraphicVisPropType=SimpleVisualProperties
  kN : Gain  Gain=1e-3
  m : Gain  Gain=1e-3
  rad/s2rpm : Gain  Gain=30/pi
  right face1 : sm_lib/Body Elements/Brick Solid  GraphicAmbientColor=[0.15 0.15 0.15 1.0]  BasedOnType=Mass  BrickDimensions=[W.pd W.pds W.pd*.5]  BrickDimensionUnits=mm  CenterOfMass=[0 0 0]  CenterOfMassUnits=m  GraphicDiffuseColor=[0.6 0.6 0.0]  Density=0  DensityUnits=g/cm^3  DoExposeReferenceFrame=on  GraphicEmissiveColor=[0.0 0.0 0.0 1.0]  ExportEntireGeometry=off  SerializedFrames=<Frames/>  MarkerShape=Sphere  MarkerSize=10  GraphicType=FromGeometry  InertiaType=CalculateFromGeometry  Mass=0  MassUnits=kg  MomentsOfInertia=[1 1 1]  MomentsOfInertiaUnits=kg*m^2  GraphicOpacity=1.0  ProductsOfInertia=[0 0 0]  ProductsOfInertiaUnits=kg*m^2  GraphicShininess=75  GraphicSpecularColor=[0.5 0.5 0.5 1.0]  GraphicVisPropType=SimpleVisualProperties
  right face2 : sm_lib/Body Elements/Brick Solid  GraphicAmbientColor=[0.15 0.15 0.15 1.0]  BasedOnType=Mass  BrickDimensions=[W.pd W.pds W.pd*.5]  BrickDimensionUnits=mm  CenterOfMass=[0 0 0]  CenterOfMassUnits=m  GraphicDiffuseColor=[0.6 0.6 0.0]  Density=0  DensityUnits=g/cm^3  DoExposeReferenceFrame=on  GraphicEmissiveColor=[0.0 0.0 0.0 1.0]  ExportEntireGeometry=off  SerializedFrames=<Frames/>  MarkerShape=Sphere  MarkerSize=10  GraphicType=FromGeometry  InertiaType=CalculateFromGeometry  Mass=0  MassUnits=kg  MomentsOfInertia=[1 1 1]  MomentsOfInertiaUnits=kg*m^2  GraphicOpacity=c.opac  ProductsOfInertia=[0 0 0]  ProductsOfInertiaUnits=kg*m^2  GraphicShininess=75  GraphicSpecularColor=[0.5 0.5 0.5 1.0]  GraphicVisPropType=SimpleVisualProperties
  rw0 : Constant  Value=W.d*0.5
  torque1 : nesl_utility/Simulink-PS Converter  PhysicalDomain=network_engine_domain  SubClassName=ps_input  LeftPortType=input  RightPortType=output  PseudoPeriodic=off  Frequencies=[]  NoiseDistribution=none  NoiseParameters=[]  Unit=N*m  AffineConversion=off  FilteringAndDerivatives=filter  SimscapeFilterOrder=2  InputFilterTimeConstant=0.001  UdotUserProvided=0
  F : PMIOPort  Side=Right
  MotSpd (rpm) : Outport  VectorParamsAs1DForOutWhenUnconnected=off
  theta [deg] : Outport  Port=2  VectorParamsAs1DForOutWhenUnconnected=off
  WinchSpd (rad/s) : Outport  Port=3  VectorParamsAs1DForOutWhenUnconnected=off
  MotTrq (Nm) : Outport  Port=4  VectorParamsAs1DForOutWhenUnconnected=off
  tag scope: S0=global, WinchAcc_L_rads=global, WinchSpd_L_rads=global, WinchTrq_L_Nm=global, w0=global
  wires:
  PS>Sim/1(Out1) -> theta [deg]/1
  Gain7/1 -> rad/s2rpm/1
  PS>Sim/9(Out9) -> [WinchSpd_L_rads], WinchSpd (rad/s)/1, Gain7/1, [w0]
  Product/1 -> Gearbox/1(MotTrq)
  Divide/1 -> kN/1
  Abs/1 -> Divide/1
  PS>Sim/4(Out4) -> Abs/1
  kN/1 -> Unit Delay1/1
  Unit Delay1/1 -> [S0]
  PS>Sim/3(Out3) -> [WinchAcc_L_rads]
  Motor/1(MotTrq) -> MotTrq (Nm)/1, Product/1
  rad/s2rpm/1 -> Gearbox/2(MotSpd), Motor/2(MotSpd), MotSpd (rpm)/1
  Product1/1 -> m/1
  m/1 -> Divide/2  "r_winch"
  winch radius/1 -> Product2/1
  rw0/1 -> Product1/2, Product2/2
  Product2/1 -> SW_wr/1
  Constant1/1 -> SW_wr/2
  SW_wr/1 -> Product/2, Product1/1
  SW_trq/1 -> Motor/1(MotTrqRef)
  MotTrqRef (Nm)/1 -> SW_trq/1
  Brake 1/1(BrkTrq) -> Add/1
  Add/1 -> [WinchTrq_L_Nm], torque1/1
  PS>Sim/2(Out2) -> Brake 1/1(speed)
  Add1/1 -> Brake 1/2(brake ON)
  Constant/1 -> Add1/1
  Brake/1 -> Add1/2
  Gearbox/2(WinchTrq') -> Add/2
  connections:
  Revolute Winch/RConn9 -- PS>Sim/LConn8
  Revolute Winch/RConn7 -- PS>Sim/LConn6
  Revolute Winch/RConn6 -- PS>Sim/LConn5
  torque1/RConn1 -- Revolute Winch/LConn2
  Revolute Winch/RConn3 -- PS>Sim/LConn2
  Revolute Winch/RConn5 -- PS>Sim/LConn4
  Revolute Winch/RConn4 -- PS>Sim/LConn3
  Revolute Winch/RConn2 -- PS>Sim/LConn1
  Revolute Winch/RConn8 -- PS>Sim/LConn7
  F/RConn1 -- Revolute Winch/RConn1
  " 2"/LConn1 -- " 4"/RConn1 -- " 6"/LConn1
  right face2/RConn1 -- " 6"/RConn1
  " 2"/RConn1 -- right face1/RConn1
  Revolute Winch/LConn1 -- Rigid Transform5/RConn1 -- " 4"/LConn1 -- " 1"/LConn1
  " 1"/RConn1 -- " "/LConn1 -- " 3"/LConn1
  " "/RConn1 -- drum end plate2/RConn1
  drum end plate1/RConn1 -- " 3"/RConn1
  World Frame/RConn1 -- Rigid Transform5/LConn1

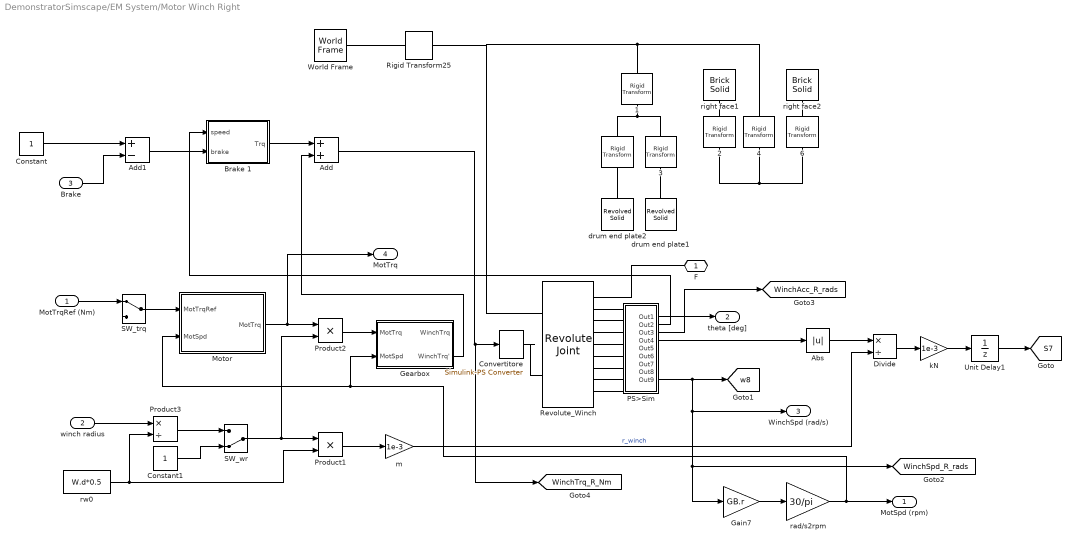
== system DemonstratorSimscape/EM System/Motor Winch Right ==
  MotTrqRef (Nm) : Inport
  winch radius : Inport  Port=2
  Brake : Inport  Port=3
  " " : sm_lib/Frames and Transforms/Rigid Transform  TranslationMethod=Cartesian  TranslationStandardOffset=0  TranslationLengthUnit=mm  TranslationStandardAxis=+Z  TranslationCartesianOffset=[0 0 -W.pds*.5]  TranslationROffset=0  TranslationROffsetUnits=m  TranslationZOffset=0  TranslationZOffsetUnits=m  TranslationThetaOffset=0  TranslationThetaOffsetUnits=deg  RotationMethod=StandardAxis  RotationAngleUnits=deg  RotationStandardAxis=-X  RotationAngle=90  RotationArbitraryAxis=[1 0 0]  FollAlignAxisA=+X  BaseAlignAxisA=+Y  FollAlignAxisB=+Y  BaseAlignAxisB=+Z  RotationSequenceAxes=FollowerAxes  RotationSequence=XYX  RotationSequenceAngles=[0 0 0]  RotationSequenceAnglesUnits=deg  RotationMatrix=[1 0 0; 0 1 0; 0 0 1]
  " 1" : sm_lib/Frames and Transforms/Rigid Transform  TranslationMethod=Cartesian  TranslationStandardOffset=0  TranslationLengthUnit=mm  TranslationStandardAxis=+Z  TranslationCartesianOffset=[0 0 W.w*0.5+W.pds*0.5]  TranslationROffset=0  TranslationROffsetUnits=m  TranslationZOffset=0  TranslationZOffsetUnits=m  TranslationThetaOffset=0  TranslationThetaOffsetUnits=deg  RotationMethod=StandardAxis  RotationAngleUnits=deg  RotationStandardAxis=+X  RotationAngle=90  RotationArbitraryAxis=[1 0 0]  FollAlignAxisA=+X  BaseAlignAxisA=+Y  FollAlignAxisB=+Y  BaseAlignAxisB=+Z  RotationSequenceAxes=FollowerAxes  RotationSequence=XYX  RotationSequenceAngles=[0 0 0]  RotationSequenceAnglesUnits=deg  RotationMatrix=[1 0 0; 0 1 0; 0 0 1]
  " 2" : sm_lib/Frames and Transforms/Rigid Transform  TranslationMethod=Cartesian  TranslationStandardOffset=0  TranslationLengthUnit=mm  TranslationStandardAxis=+Z  TranslationCartesianOffset=[0 -W.pd*.25 -W.pds]  TranslationROffset=0  TranslationROffsetUnits=m  TranslationZOffset=0  TranslationZOffsetUnits=m  TranslationThetaOffset=0  TranslationThetaOffsetUnits=deg  RotationMethod=ArbitraryAxis  RotationAngleUnits=deg  RotationStandardAxis=+X  RotationAngle=90  RotationArbitraryAxis=[1 0 0]  FollAlignAxisA=+X  BaseAlignAxisA=+Y  FollAlignAxisB=+Y  BaseAlignAxisB=+Z  RotationSequenceAxes=FollowerAxes  RotationSequence=XYX  RotationSequenceAngles=[0 0 0]  RotationSequenceAnglesUnits=deg  RotationMatrix=[1 0 0; 0 1 0; 0 0 1]
  " 3" : sm_lib/Frames and Transforms/Rigid Transform  TranslationMethod=Cartesian  TranslationStandardOffset=0  TranslationLengthUnit=mm  TranslationStandardAxis=+Z  TranslationCartesianOffset=[0 -W.w -W.pds*.5]  TranslationROffset=0  TranslationROffsetUnits=m  TranslationZOffset=0  TranslationZOffsetUnits=m  TranslationThetaOffset=0  TranslationThetaOffsetUnits=deg  RotationMethod=StandardAxis  RotationAngleUnits=deg  RotationStandardAxis=+X  RotationAngle=90  RotationArbitraryAxis=[1 0 0]  FollAlignAxisA=+X  BaseAlignAxisA=+Y  FollAlignAxisB=+Y  BaseAlignAxisB=+Z  RotationSequenceAxes=FollowerAxes  RotationSequence=XYX  RotationSequenceAngles=[0 0 0]  RotationSequenceAnglesUnits=deg  RotationMatrix=[1 0 0; 0 1 0; 0 0 1]
  " 4" : sm_lib/Frames and Transforms/Rigid Transform  TranslationMethod=Cartesian  TranslationStandardOffset=0  TranslationLengthUnit=mm  TranslationStandardAxis=+Z  TranslationCartesianOffset=[0 0 -W.w*.5]  TranslationROffset=0  TranslationROffsetUnits=m  TranslationZOffset=0  TranslationZOffsetUnits=m  TranslationThetaOffset=0  TranslationThetaOffsetUnits=deg  RotationMethod=None  RotationAngleUnits=deg  RotationStandardAxis=+Z  RotationAngle=90  RotationArbitraryAxis=[1 0 0]  FollAlignAxisA=+X  BaseAlignAxisA=+Y  FollAlignAxisB=+Y  BaseAlignAxisB=+Z  RotationSequenceAxes=FollowerAxes  RotationSequence=XYX  RotationSequenceAngles=[0 0 0]  RotationSequenceAnglesUnits=deg  RotationMatrix=[1 0 0; 0 1 0; 0 0 1]
  " 6" : sm_lib/Frames and Transforms/Rigid Transform  TranslationMethod=Cartesian  TranslationStandardOffset=0  TranslationLengthUnit=mm  TranslationStandardAxis=+Z  TranslationCartesianOffset=[0 -W.pd*.25 W.w+W.pds*2]  TranslationROffset=0  TranslationROffsetUnits=m  TranslationZOffset=0  TranslationZOffsetUnits=m  TranslationThetaOffset=0  TranslationThetaOffsetUnits=deg  RotationMethod=ArbitraryAxis  RotationAngleUnits=deg  RotationStandardAxis=+X  RotationAngle=90  RotationArbitraryAxis=[1 0 0]  FollAlignAxisA=+X  BaseAlignAxisA=+Y  FollAlignAxisB=+Y  BaseAlignAxisB=+Z  RotationSequenceAxes=FollowerAxes  RotationSequence=XYX  RotationSequenceAngles=[0 0 0]  RotationSequenceAnglesUnits=deg  RotationMatrix=[1 0 0; 0 1 0; 0 0 1]
  Abs : Abs
  Add : Sum
  Add1 : Sum  Inputs=+-
  Brake 1 : Subsystem
  Constant : Constant
  Constant1 : Constant
  Convertitore : nesl_utility/Simulink-PS Converter  PhysicalDomain=network_engine_domain  SubClassName=ps_input  LeftPortType=input  RightPortType=output  PseudoPeriodic=off  Frequencies=[]  NoiseDistribution=none  NoiseParameters=[]  Unit=1  AffineConversion=off  FilteringAndDerivatives=filter  SimscapeFilterOrder=2  InputFilterTimeConstant=0.001  UdotUserProvided=2
  Divide : Product  Inputs=*/
  Gain7 : Gain  Gain=GB.r
  Gearbox : Subsystem
  Motor : Subsystem
  PS>Sim : Subsystem
  Product1 : Product
  Product2 : Product
  Product3 : Product  Inputs=*/
  Revolute_Winch : sm_lib/Joints/Revolute Joint  JointMode=Normal  SenseConstraintForce=on  SenseConstraintForceX=off  SenseConstraintForceY=off  SenseConstraintForceZ=off  SenseConstraintTorque=on  SenseConstraintTorqueX=off  SenseConstraintTorqueY=off  SenseConstraintTorqueZ=off  SenseTotalForce=on  SenseTotalForceX=off  SenseTotalForceY=off  SenseTotalForceZ=off  SenseTotalTorque=on  SenseTotalTorqueX=off  SenseTotalTorqueY=off  SenseTotalTorqueZ=off  CompositeWrenchDir=FollowerOnBase  CompositeWrenchFrame=BaseFrame  EquilibriumPosition=0  EquilibriumPositionUnits=deg  SpringStiffness=0  SpringStiffnessUnits=N*m/deg  DampingCoefficient=b_winch  DampingCoefficientUnits=N*m/(deg/s)  TorqueActuationMode=InputTorque  MotionActuationMode=ComputedMotion  SensePosition=on  SenseVelocity=on  SenseAcceleration=on  SenseTorqueForce=on  SenseLowerLimitTorqueForce=off  SenseUpperLimitTorqueForce=off  LowerLimitSpecify=off  LowerLimitBound=-90  LowerLimitBoundUnits=deg  LowerLimitStiffness=1e4  LowerLimitStiffnessUnits=N*m/deg  LowerLimitDamping=10  LowerLimitDampingUnits=N*m/(deg/s)  LowerLimitTransitionRegionWidth=0.1  LowerLimitTransitionRegionWidthUnits=deg  UpperLimitSpecify=off  UpperLimitBound=90  UpperLimitBoundUnits=deg  UpperLimitStiffness=1e4  UpperLimitStiffnessUnits=N*m/deg  UpperLimitDamping=10  UpperLimitDampingUnits=N*m/(deg/s)  UpperLimitTransitionRegionWidth=0.1  UpperLimitTransitionRegionWidthUnits=deg  PositionTargetSpecify=off  PositionTargetPriority=High  PositionTargetValue=0  PositionTargetValueUnits=deg  VelocityTargetSpecify=on  VelocityTargetPriority=High  VelocityTargetValue=w0_winch  VelocityTargetValueUnits=deg/s
  Rigid Transform25 : sm_lib/Frames and Transforms/Rigid Transform  TranslationMethod=Cartesian  TranslationStandardOffset=0  TranslationLengthUnit=mm  TranslationStandardAxis=+Z  TranslationCartesianOffset="[0.5*T.s2+0.5*W.d  W.pd*.5  0]"  TranslationROffset=0  TranslationROffsetUnits=m  TranslationZOffset=0  TranslationZOffsetUnits=m  TranslationThetaOffset=0  TranslationThetaOffsetUnits=deg  RotationMethod=None  RotationAngleUnits=deg  RotationStandardAxis=+Z  RotationAngle=0.0  RotationArbitraryAxis=[0 0 1]  FollAlignAxisA=+X  BaseAlignAxisA=+Y  FollAlignAxisB=+Y  BaseAlignAxisB=+Z  RotationSequenceAxes=FollowerAxes  RotationSequence=XYX  RotationSequenceAngles=[0 0 0]  RotationSequenceAnglesUnits=deg  RotationMatrix=[1 0 0; 0 1 0; 0 0 1]
  SW_trq : ManualSwitch
  SW_wr : ManualSwitch  CurrentSetting=0
  Unit Delay1 : UnitDelay  InitialCondition=130.83  SampleTime=-1  HasFrameUpgradeWarning=on
  World Frame : sm_lib/Frames and Transforms/World Frame
  drum end plate1 : sm_lib/Body Elements/Revolved Solid  GraphicAmbientColor=[0.15 0.15 0.15 1.0]  BasedOnType=Density  CenterOfMass=[0 0 0]  CenterOfMassUnits=m  GraphicDiffuseColor=[1.0 0.2 0.2]  ExportConvexHullGeometry=off  Density=0  DensityUnits=g/cm^3  DoExposeReferenceFrame=on  GraphicEmissiveColor=[0.0 0.0 0.0 1.0]  ExportEntireGeometry=off  SerializedFrames=<Frames/>  MarkerShape=Sphere  MarkerSize=10  GraphicType=FromGeometry  InertiaType=CalculateFromGeometry  Mass=1  MassUnits=kg  MomentsOfInertia=[1 1 1]  MomentsOfInertiaUnits=kg*m^2  GraphicOpacity=1.0  ProductsOfInertia=[0 0 0]  ProductsOfInertiaUnits=kg*m^2  RevolutionCrossSection=[W.pd*.5 0; W.pd*.5 W.pds; W.pd*0.05 W.pds; W.pd*.05 0]  RevolutionCrossSectionUnits=mm  RevolutionAngle=180  RevolutionAngleUnits=deg  RevolutionExtent=Full  GraphicShininess=75  GraphicSpecularColor=[0.5 0.5 0.5 1.0]  GraphicVisPropType=SimpleVisualProperties
  drum end plate2 : sm_lib/Body Elements/Revolved Solid  GraphicAmbientColor=[0.15 0.15 0.15 1.0]  BasedOnType=Density  CenterOfMass=[0 0 0]  CenterOfMassUnits=m  GraphicDiffuseColor=[0.0 0.8 0.0]  ExportConvexHullGeometry=off  Density=0  DensityUnits=g/cm^3  DoExposeReferenceFrame=on  GraphicEmissiveColor=[0.0 0.0 0.0 1.0]  ExportEntireGeometry=off  SerializedFrames=<Frames/>  MarkerShape=Sphere  MarkerSize=10  GraphicType=FromGeometry  InertiaType=CalculateFromGeometry  Mass=1  MassUnits=kg  MomentsOfInertia=[1 1 1]  MomentsOfInertiaUnits=kg*m^2  GraphicOpacity=1.0  ProductsOfInertia=[0 0 0]  ProductsOfInertiaUnits=kg*m^2  RevolutionCrossSection=[W.pd*.5 0; W.pd*.5 W.pds; W.pd*0.05 W.pds; W.pd*.05 0]  RevolutionCrossSectionUnits=mm  RevolutionAngle=180  RevolutionAngleUnits=deg  RevolutionExtent=Full  GraphicShininess=75  GraphicSpecularColor=[0.5 0.5 0.5 1.0]  GraphicVisPropType=SimpleVisualProperties
  kN : Gain  Gain=1e-3
  m : Gain  Gain=1e-3
  rad/s2rpm : Gain  Gain=30/pi
  right face1 : sm_lib/Body Elements/Brick Solid  GraphicAmbientColor=[0.15 0.15 0.15 1.0]  BasedOnType=Mass  BrickDimensions=[W.pd W.pds W.pd*.5]  BrickDimensionUnits=mm  CenterOfMass=[0 0 0]  CenterOfMassUnits=m  GraphicDiffuseColor=[0.6 0.6 0.0]  Density=0  DensityUnits=g/cm^3  DoExposeReferenceFrame=on  GraphicEmissiveColor=[0.0 0.0 0.0 1.0]  ExportEntireGeometry=off  SerializedFrames=<Frames/>  MarkerShape=Sphere  MarkerSize=10  GraphicType=FromGeometry  InertiaType=CalculateFromGeometry  Mass=0  MassUnits=kg  MomentsOfInertia=[1 1 1]  MomentsOfInertiaUnits=kg*m^2  GraphicOpacity=1.0  ProductsOfInertia=[0 0 0]  ProductsOfInertiaUnits=kg*m^2  GraphicShininess=75  GraphicSpecularColor=[0.5 0.5 0.5 1.0]  GraphicVisPropType=SimpleVisualProperties
  right face2 : sm_lib/Body Elements/Brick Solid  GraphicAmbientColor=[0.15 0.15 0.15 1.0]  BasedOnType=Mass  BrickDimensions=[W.pd W.pds W.pd*.5]  BrickDimensionUnits=mm  CenterOfMass=[0 0 0]  CenterOfMassUnits=m  GraphicDiffuseColor=[0.6 0.6 0.0]  Density=0  DensityUnits=g/cm^3  DoExposeReferenceFrame=on  GraphicEmissiveColor=[0.0 0.0 0.0 1.0]  ExportEntireGeometry=off  SerializedFrames=<Frames/>  MarkerShape=Sphere  MarkerSize=10  GraphicType=FromGeometry  InertiaType=CalculateFromGeometry  Mass=0  MassUnits=kg  MomentsOfInertia=[1 1 1]  MomentsOfInertiaUnits=kg*m^2  GraphicOpacity=c.opac  ProductsOfInertia=[0 0 0]  ProductsOfInertiaUnits=kg*m^2  GraphicShininess=75  GraphicSpecularColor=[0.5 0.5 0.5 1.0]  GraphicVisPropType=SimpleVisualProperties
  rw0 : Constant  Value=W.d*0.5
  F : PMIOPort  Side=Right
  MotSpd (rpm) : Outport  VectorParamsAs1DForOutWhenUnconnected=off
  theta [deg] : Outport  Port=2  VectorParamsAs1DForOutWhenUnconnected=off
  WinchSpd (rad/s) : Outport  Port=3  VectorParamsAs1DForOutWhenUnconnected=off
  MotTrq : Outport  Port=4  VectorParamsAs1DForOutWhenUnconnected=off
  tag scope: S7=global, WinchAcc_R_rads=global, WinchSpd_R_rads=global, WinchTrq_R_Nm=global, w8=global
  wires:
  PS>Sim/1(Out1) -> theta [deg]/1
  PS>Sim/4(Out4) -> Abs/1
  Product2/1 -> Gearbox/1(MotTrq)
  Gain7/1 -> rad/s2rpm/1
  PS>Sim/9(Out9) -> [WinchSpd_R_rads], Gain7/1, WinchSpd (rad/s)/1, [w8]
  Abs/1 -> Divide/1
  Divide/1 -> kN/1
  kN/1 -> Unit Delay1/1
  Unit Delay1/1 -> [S7]
  PS>Sim/3(Out3) -> [WinchAcc_R_rads]
  SW_trq/1 -> Motor/1(MotTrqRef)
  Motor/1(MotTrq) -> MotTrq/1, Product2/1
  rad/s2rpm/1 -> Gearbox/2(MotSpd), Motor/2(MotSpd), MotSpd (rpm)/1
  Product1/1 -> m/1
  rw0/1 -> Product1/2, Product3/2
  SW_wr/1 -> Product2/2, Product1/1
  Constant1/1 -> SW_wr/2
  winch radius/1 -> Product3/1
  Product3/1 -> SW_wr/1
  m/1 -> Divide/2  "r_winch"
  MotTrqRef (Nm)/1 -> SW_trq/1
  Brake 1/1(Trq) -> Add/1
  Gearbox/2(WinchTrq') -> Add/2
  Add/1 -> [WinchTrq_R_Nm], Convertitore/1
  PS>Sim/2(Out2) -> Brake 1/1(speed)
  Add1/1 -> Brake 1/2(brake)
  Brake/1 -> Add1/2
  Constant/1 -> Add1/1
  connections:
  Revolute_Winch/RConn4 -- PS>Sim/LConn3
  Revolute_Winch/RConn2 -- PS>Sim/LConn1
  " 1"/LConn1 -- Revolute_Winch/LConn1 -- Rigid Transform25/RConn1 -- " 4"/LConn1
  " 2"/LConn1 -- " 6"/LConn1 -- " 4"/RConn1
  right face2/RConn1 -- " 6"/RConn1
  " 2"/RConn1 -- right face1/RConn1
  drum end plate1/RConn1 -- " 3"/RConn1
  " "/RConn1 -- drum end plate2/RConn1
  " "/LConn1 -- " 3"/LConn1 -- " 1"/RConn1
  Revolute_Winch/RConn3 -- PS>Sim/LConn2
  Revolute_Winch/RConn5 -- PS>Sim/LConn4
  Revolute_Winch/RConn6 -- PS>Sim/LConn5
  Revolute_Winch/RConn7 -- PS>Sim/LConn6
  Revolute_Winch/RConn8 -- PS>Sim/LConn7
  Revolute_Winch/RConn9 -- PS>Sim/LConn8
  F/RConn1 -- Revolute_Winch/RConn1
  Convertitore/RConn1 -- Revolute_Winch/LConn2
  World Frame/RConn1 -- Rigid Transform25/LConn1
